simulink model "HWCOSIM_PHcontr_V2"  (R2020a)
settings: Solver=ode45  StartTime=0.0  StopTime=20  MaxStep=1e-5  RelTol=1e-3
undefined symbols (not defined in the file): A, den_loop_filtZ, f_step, fdesignblkfcn, FPGA_CLK, FPGA_Ts, Fref, G_loopfilt, gcbh, max_unwrap_periods, MECOS_cl_den, MECOS_MAX_PULSES, N, Nslits, num_loop_filtZ, PFD_noise_corrtime, PFD_Ts, phase_setpoint_degrees, PHCTRLR_CLK, PHCTRLR_Ts, Tref, unwrap_res_thr
libraries: dspsigops x5, simulink x4, dspmlti4 x4, simulink_extras x2, xbsIndex_r4 x1, dsparch4 x1, dspfdesign x1, JTAGRuntimeCosim_r4 x1
settings Model: Creator=valbas  LastModifiedBy=valbas
settings SolverCC: AlgebraicLoopSolver=LineSearch

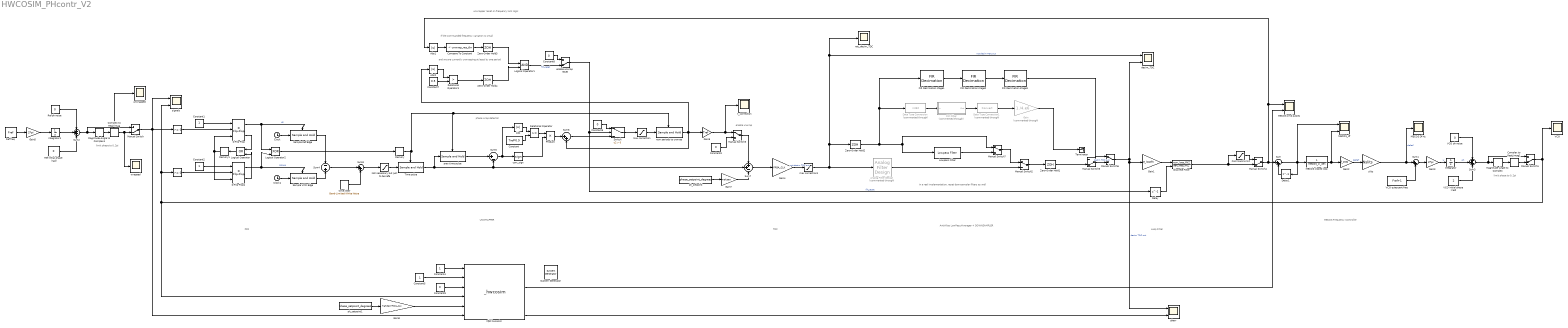
== system HWCOSIM_PHcontr_V2 ==
  note: enable unwrap
  note: in a real implementation, reset downsampler filters as well
  note: if the commanded frequency variation is small
  note: unwrapper reset on frequency lock logic
  note: phase wrap detector
  note: limit phase to 0..2pi
  note: TDC
  note: AntiAlias LowPass/Averager +
      | DOWNSAMPLER
  note: Loop Filter
  note: MECOS Frequency Controller
  note: limit phase to 0..2pi
  note: PFD
  note: UNWRAPPER
  note: and we are currently unwrapping at least by one period
  " " : simulink/Logic and Bit Operations/Compare To Constant  relop=>=  const=0  OutDataTypeStr=boolean
  "  " : simulink/Logic and Bit Operations/Compare To Constant  relop=>=  const=0  OutDataTypeStr=boolean
  " System Generator" : xbsIndex_r4/ System Generator  Tag=genX  xilinxfamily=zynq  part=xc7z020  speed=-1  package=clg484  synthesis_tool=Vivado  clock_wrapper=Clock Enables  directory=./netlist  proj_type=Vivado  Synth_file=Vivado Synthesis Defaults  Impl_file=Vivado Implementation Defaults  testbench=off  simulink_period=FPGA_Ts  sysclk_period=FPGA_Ts*1e9  dcm_input_clock_period=10  incr_netlist=off  trim_vbits=Everywhere in SubSystem  dbl_ovrd=According to Block Masks  core_generation=According to Block Masks  run_coregen=off  deprecated_control=off  eval_field=0  block_type=sysgen
  Abs : Abs
  Abs1 : Abs
  Abs2 : Abs
  Analog Filter Design : dsparch4/Analog Filter Design  Commented=through  method=Chebyshev II  filttype=Lowpass  N=8  Wlo=100  Whi=80  Rp=2  Rs=50
  CIC Filter : Subsystem  Commented=through  DialogController=fdesignblkfcn  InitFcn=fdesignblkfcn(gcbh, {'InitFcn'});  mask(CIC Filter){}
      mask help: Design a CIC filter
      settings: CopyFcn=fdesignblkfcn(gcbh, {'CopyFcn'});
      mask Help: helpview(mapfilelocation('dsp'), 'dspcicfilter');
      mask Display: disp('CIC')
  Clock : Clock
  Clock1 : Clock
  Command Limit : Saturate  UpperLimit=MECOS_MAX_PULSES/PHCTRLR_CLK  LowerLimit=-MECOS_MAX_PULSES/PHCTRLR_CLK
  Compare To Constant : simulink/Logic and Bit Operations/Compare To Constant  relop=<  const=unwrap_res_thr  OutDataTypeStr=boolean
  Complex to Real-Imag : ComplexToRealImag  Output=Real
  Complex to Real-Imag1 : ComplexToRealImag  Output=Real
  Constant : Constant  Value=Tref*0.9
  Constant{1..2,4..5} (4 alike) : Constant  OutDataTypeStr=boolean
  Constant3 : Constant  Value=0
  Constant6 : Constant  Value=0
  Constant7 : Constant  Value=0.5
  Constant8 : Constant  Value=0  OutDataTypeStr=boolean
  Constant9 : Constant  Value=0  OutDataTypeStr=boolean
  D Flip-Flop : simulink_extras/Flip Flops/D Flip-Flop
  D Flip-Flop1 : simulink_extras/Flip Flops/D Flip-Flop
  Data Type Conversion : DataTypeConversion  Commented=through  OutDataTypeStr=int32  RndMeth=Round
  Data Type Conversion1 : DataTypeConversion  Commented=through  RndMeth=Round
  Delay : Delay  DelayLength=1
  Delay1 : Delay  DelayLength=1
  Discrete Filter : DiscreteFilter  Numerator=num_loop_filtZ  Denominator=den_loop_filtZ  ExternalReset=Rising
      settings: InputPortMap=u0,r7
  FIR Decimation stage1 : dspmlti4/FIR Decimation  FilterSource=Dialog parameters  h=Num  D=10  filtStruct=Direct form  FilterObject=FDECIM  InputProcessing=Columns as channels (frame based)  framing=Allow multirate processing  inputOffset=0  outputBufInitCond=0  roundingMode=Floor  overflowMode=off  firstCoeffDataTypeStr=Inherit: Same word length as input  firstCoeffMin=[]  firstCoeffMax=[]  firstCoeffLastDataTypeStr=Inherit: Same word length as input  outputDataTypeStr=Inherit: Same as accumulator  outputMin=[]  outputMax=[]  outputLastDataTypeStr=Inherit: Same as accumulator
  FIR Decimation stage2 : dspmlti4/FIR Decimation  FilterSource=Dialog parameters  h=Num  D=10  filtStruct=Direct form  FilterObject=FDECIM  InputProcessing=Columns as channels (frame based)  framing=Allow multirate processing  inputOffset=0  outputBufInitCond=0  roundingMode=Floor  overflowMode=off  firstCoeffDataTypeStr=Inherit: Same word length as input  firstCoeffMin=[]  firstCoeffMax=[]  firstCoeffLastDataTypeStr=Inherit: Same word length as input  outputDataTypeStr=Inherit: Same as accumulator  outputMin=[]  outputMax=[]  outputLastDataTypeStr=Inherit: Same as accumulator
  FIR Decimation stage3 : dspmlti4/FIR Decimation  FilterSource=Dialog parameters  h=Num  D=10  filtStruct=Direct form  FilterObject=FDECIM  InputProcessing=Columns as channels (frame based)  framing=Allow multirate processing  inputOffset=0  outputBufInitCond=0  roundingMode=Floor  overflowMode=off  firstCoeffDataTypeStr=Inherit: Same word length as input  firstCoeffMin=[]  firstCoeffMax=[]  firstCoeffLastDataTypeStr=Inherit: Same word length as input  outputDataTypeStr=Inherit: Same as accumulator  outputMin=[]  outputMax=[]  outputLastDataTypeStr=Inherit: Same as accumulator
  Gain : Gain  Commented=through  Gain=1./4.e6
  Gain1 : Gain  Gain=G_loopfilt
  Gain2 : Gain  Gain=f_step
  Gain3 : Gain  Gain=2*pi
  Gain4 : Gain  Gain=FPGA_CLK
  Gain5 : Gain  Gain=2*pi
  Gain6 : Gain  Gain=Tref
  Gain7 : Gain  Gain=Tref/360
  Gain8 : Gain  Gain=Tref/360*FPGA_CLK
  Integrator : Integrator
  Integrator1 : Integrator
  Logical Operator : Logic  Operator=OR  IconShape=distinctive  AllPortsSameDT=off  OutDataTypeStr=boolean
  Logical Operator1 : Logic  IconShape=distinctive  AllPortsSameDT=off  OutDataTypeStr=boolean
  Logical Operator2 : Logic  Operator=XOR  IconShape=distinctive  AllPortsSameDT=off  OutDataTypeStr=boolean
  Lowpass Filter : dspfdesign/Lowpass Filter  FilterType=FIR  DesignForMinimumOrder=on  FilterOrder=50  PassbandFrequency=30  StopbandFrequency=70  PassbandRipple=1  StopbandAttenuation=30  InheritSampleRate=off  SampleRate=100e3  SimulateUsing=Interpreted execution  roundingMode=Floor  coeffsDataTypeStr=fixdt(1,16)
  MECOS Df Hz : Scope
  MECOS closed loop : TransferFcn  Denominator=MECOS_cl_den
  MECOS cmd pulses : Scope  NumInputPorts=2
  MECOS_df : Scope  NumInputPorts=2
  Magnitude-Angle to Complex : MagnitudeAngleToComplex  Input=Angle  ConstantPart=1
  Magnitude-Angle to Complex1 : MagnitudeAngleToComplex  Input=Angle  ConstantPart=1
  Manual Switch{,1,4..5} (4 alike) : ManualSwitch  CurrentSetting=0
  Manual Switch{2..3,6..7} (4 alike) : ManualSwitch
  Memory : Memory
  Memory1 : Memory
  Not necessary but just to be safe : Saturate  UpperLimit=Tref  LowerLimit=-Tref
  Product : Product
  Ref freq : Constant  Value=Fref
  Ref initial phase (rad) : Constant  Value=0
  Ref ph noise : Constant  Value=0
  Relational Operator : RelationalOperator  OutDataTypeStr=boolean  RndMeth=Simplest
  Relational Operator1 : RelationalOperator  Operator=>  OutDataTypeStr=boolean  RndMeth=Simplest
  Sample Ref Edge : dspsigops/Sample and Hold  trig=Rising edge  initCond=0  latchinput=on
  Sample VCO Edge : dspsigops/Sample and Hold  trig=Rising edge  initCond=0  latchinput=on
  Sum{,1,6,8} (4 alike) : Sum  Inputs=|++
  Sum2 : Sum  Inputs=+++
  Sum3 : Sum  Inputs=+++
  Sum4 : Sum  Inputs=-|+
  Sum5 : Sum  Inputs=|+-
  Sum7 : Sum  Inputs=++-
  Switch : Switch  Criteria=u2 > Threshold
  Terminator : Terminator
  Time pulse : dspsigops/Sample and Hold  trig=Falling edge  initCond=0  latchinput=on
  VCO : Scope
  VCO initial phase (rad) : Constant  Value=2
  VCO ph noise : Constant  Value=0
  VCO quiescent freq : Constant  Value=Fref+1
  Zero-Order Hold1 : ZeroOrderHold  SampleTime=PHCTRLR_Ts
  Zero-Order Hold2 : ZeroOrderHold  SampleTime=PFD_Ts
  Zero-Order Hold3 : ZeroOrderHold  SampleTime=PHCTRLR_Ts
  Zero-Order Hold4 : ZeroOrderHold  SampleTime=PHCTRLR_Ts
  corr_sign : Signum
  decim_TDC : Scope  NumInputPorts=2
  enable unwrap reset : ManualSwitch  CurrentSetting=0
  max correction : Saturate  UpperLimit=max_unwrap_periods  LowerLimit=-max_unwrap_periods
  max correction1 : Saturate  UpperLimit=max_unwrap_periods*Tref*FPGA_CLK  LowerLimit=-max_unwrap_periods*Tref*FPGA_CLK
  not_decim_TDC : Scope
  num periods to unwrap : dspsigops/Sample and Hold  trig=Falling edge  initCond=0  latchinput=on
  ph_setpoint : Constant  Value=phase_setpoint_degrees
  ph_setpoint1 : Constant  Value=phase_setpoint_degrees
  pherr : Scope  NumInputPorts=2
  prev time pulse : dspsigops/Sample and Hold  trig=Falling edge  initCond=0  latchinput=on
  signals : Scope  NumInputPorts=2
  slits : Gain  Gain=Nslits
  t_correction : Scope
  time jitter : simulink/Sources/Band-Limited White Noise  Cov=PFD_jitter_PSD  Ts=PFD_noise_corrtime  seed=[23341]
  unwrapped : Scope
  wrapped : Scope
  zfph hwcosim : JTAGRuntimeCosim_r4/_hwcosim  clkSrc=Single Stepped  hasCombinationalPath=on  bitfileName=C:\xilinxworks\netlist\zfph.bit  skipConfig=off  dispPartInfo=off  useZynqReconfigScript=on  cable=Auto Detect  speed=N/A  cablePort=N/A  cableLocation=Local  shareCable=off  design_xtable=|  engineDll=JTAGCosimEngine.dll  cableWaitTime=10  bscanPos=-1  IRLengths=[]  useWaitBox=1  hasBufgmux=on  Scheme=Cosim  useCmdProc=1  hasProc=0  useImpact=0  printLogFile=0  userChain=2  block_type=jtagcosim
      | {
      |     'clkWrapper' => 'zfph',
      |     'burstMode' => false,
      |     'burstFifoDepth' => '1024',
      |     'shared_memories' => {},
      |     'clocksGcd' => 1,
      |     'device' => {
      |       'family' => 'zynq',
      |       'part' => 'xc7z020',
      |       'package' => 'clg484',
      |       'speed' => '-1',
      |     },
      |     'ports' => {
      |       'unwr_reset_enable' => {
      |         'direction' => 'in',
      |         'width' => 1,
      |         'name' => 'unwr_reset_enable',
      |         'period' => 1,
      |         'icon_text' => 'unwr_reset_enable',
      |         'type' => 'Bool',
      |         'arithmetic_type' => 'xlUnsigned',
      |         'dat_file' => 'zfph_unwr_reset_enable.dat',
      |         'bin_pt' => 0,
      |         'addr_offset' => 0,
      |         'bd_port_index' => 0,
      |       },
      |       'unwr_en' => {
      |         'direction' => 'in',
      |         'width' => 1,
      |         'name' => 'unwr_en',
      |         'period' => 1,
      |         'icon_text' => 'unwr_en',
      |         'type' => 'Bool',
      |         'arithmetic_type' => 'xlUnsigned',
      |         'dat_file' => 'zfph_unwr_en.dat',
      |         'bin_pt' => 0,
      |         'addr_offset' => 4,
      |         'bd_port_index' => 1,
      |       },
      |       'reset' => {
      |         'direction' => 'in',
      |         'width' => 1,
      |         'name' => 'reset',
      |         'period' => 1,
      |         'icon_text' => 'reset',
      |         'type' => 'Bool',
      |         'arithmetic_type' => 'xlUnsigned',
      |         'dat_file' => 'zfph_reset.dat',
      |         'bin_pt' => 0,
      |         'addr_offset' => 8,
      |         'bd_port_index' => 2,
      |       },
      |       'vcoin' => {
      |         'direction' => 'in',
      |         'width' => 1,
      |         'name' => 'vcoin',
      |         'period' => 1,
      |         'icon_text' => 'VCOin',
      |         'type' => 'Bool',
      |         'arithmetic_type' => 'xlUnsigned',
      |         'dat_file' => 'zfph_vcoin.dat',
      |         'bin_pt' => 0,
      |         'addr_offset' => 12,
      |         'bd_port_index' => 3,
      |       },
      |       'setpoint_cnts' => {
      |         'direction' => 'in',
      |         'width' => 17,
      |         'name' => 'setpoint_cnts',
      |         'period' => 1,
      |         'icon_text' => 'Setpoint_cnts',
      |         'type' => 'Fix_17_0',
      |         'arithmetic_type' => 'xlSigned',
      |         'dat_file' => 'zfph_setpoint_cnts.dat',
      |         'bin_pt' => 0,
      |         'addr_offset' => 16,
      |         'bd_port_index' => 4,
      |       },
      |       'refin' => {
      |         'direction' => 'in',
      |         'width' => 1,
      |         'name' => 'refin',
      |         'period' => 1,
      |         'icon_text' => 'REFin',
      |         'type' => 'Bool',
      |         'arithmetic_type' => 'xlUnsigned',
      |         'dat_file' => 'zfph_refin.dat',
      |         'bin_pt' => 0,
      |         'addr_offset' => 20,
      |         'bd_port_index' => 5,
      |       },
      |       'dec_pulses' => {
      |         'direction' => 'out',
      |         'width' => 1,
      |         'name' => 'dec_pulses',
      |         'period' => 12500,
      |         'icon_text' => 'DEC_PULSES',
      |         'type' => 'Bool',
      |         'arithmetic_type' => 'xlUnsigned',
      |         'dat_file' => 'zfph_dec_pulses.dat',
      |         'bin_pt' => 0,
      |         'addr_offset' => 24,
      |         'bd_port_index' => 0,
      |       },
      |       'dec_pwm' => {
      |         'direction' => 'out',
      |         'width' => 1,
      |         'name' => 'dec_pwm',
      |         'period' => 12500,
      |         'icon_text' => 'DEC_PWM',
      |         'type' => 'Bool',
      |         'arithmetic_type' => 'xlUnsigned',
      |         'dat_file' => 'zfph_dec_pwm.dat',
      |         'bin_pt' => 0,
      |         'addr_offset' => 28,
      |         'bd_port_index' => 1,
      |       },
      |       'df_comm' => {
      |         'direction' => 'out',
      |         'width' => 22,
      |         'name' => 'df_comm',
      |         'period' => 1250000,
      |         'icon_text' => 'DF_COMM',
      |         'type' => 'Fix_22_0',
      |         'arithmetic_type' => 'xlSigned',
      |         'dat_file' => 'zfph_df_comm.dat',
      |         'bin_pt' => 0,
      |         'addr_offset' => 32,
      |         'bd_port_index' => 2,
      |       },
      |       'inc_pulses' => {
      |         'direction' => 'out',
      |         'width' => 1,
      |         'name' => 'inc_pulses',
      |         'period' => 12500,
      |         'icon_text' => 'INC_PULSES',
      |         'type' => 'Bool',
      |         'arithmetic_type' => 'xlUnsigned',
      |         'dat_file' => 'zfph_inc_pulses.dat',
      |         'bin_pt' => 0,
      |         'addr_offset' => 36,
      |         'bd_port_index' => 3,
      |       },
      |       'inc_pwm' => {
      |         'direction' => 'out',
      |         'width' => 1,
      |         'name' => 'inc_pwm',
      |         'period' => 12500,
      |         'icon_text' => 'INC_PWM',
      |         'type' => 'Bool',
      |         'arithmetic_type' => 'xlUnsigned',
      |         'dat_file' => 'zfph_inc_pwm.dat',
      |         'bin_pt' => 0,
      |         'addr_offset' => 40,
      |         'bd_port_index' => 4,
      |       },
      |       'ph_err' => {
      |         'direction' => 'out',
      |         'width' => 24,
      |         'name' => 'ph_err',
      |         'period' => 1250000,
      |         'icon_text' => 'PH_ERR',
      |         'type' => 'Fix_24_7',
      |         'arithmetic_type' => 'xlSigned',
      |         'dat_file' => 'zfph_ph_err.dat',
      |         'bin_pt' => 7,
      |         'addr_offset' => 44,
      |         'bd_port_index' => 5,
      |       },
      |     },
      |   }
  wires:
  Gain1/1 -> Discrete Filter/1
  Manual Switch6/1 -> decim_TDC/2, pherr/1, Gain1/1  "decim TDC out"
  Delay1/1 -> Sum/2
  Sum/1 -> Delay1/1, MECOS closed loop/1, MECOS_df/1
  MECOS closed loop/1 -> Gain2/1, MECOS_df/2
  slits/1 -> MECOS Df Hz/1, Sum1/1  "deltaf"
  VCO quiescent freq/1 -> Sum1/2
  Sum1/1 -> Gain3/1
  Gain3/1 -> Integrator/1  "w"
  Integrator/1 -> Sum3/2  "ph"
  Magnitude-Angle to Complex/1 -> Complex to Real-Imag1/1
  Magnitude-Angle to Complex1/1 -> Complex to Real-Imag/1
  Gain5/1 -> Integrator1/1
  Ref freq/1 -> Gain5/1
  VCO initial phase (rad)/1 -> Sum3/3
  Sum3/1 -> Manual Switch1/1, Magnitude-Angle to Complex/1
  Sum2/1 -> unwrapped/1, Manual Switch/1, Magnitude-Angle to Complex1/1
  Complex to Real-Imag/1 -> wrapped/1, Manual Switch/2
  max correction1/1 -> not_decim_TDC/1, decim_TDC/1, Zero-Order Hold2/1, Analog Filter Design/1  "not decim TDC out"
  Manual Switch/1 -> zfph hwcosim/6, signals/1, " "/1
  Complex to Real-Imag1/1 -> Manual Switch1/2
  Discrete Filter/1 -> Command Limit/1, Manual Switch4/2
  Lowpass Filter/1 -> Manual Switch7/2
  Analog Filter Design/1 -> Manual Switch2/2
  Manual Switch2/1 -> Zero-Order Hold1/1
  " "/1 -> D Flip-Flop/2
  Sample Ref Edge/1 -> Sum4/1
  "  "/1 -> D Flip-Flop1/2
  Manual Switch1/1 -> VCO/1, "  "/1, signals/2, zfph hwcosim/4
  Sample VCO Edge/1 -> Sum4/2
  Clock/1 -> Sample Ref Edge/1
  Clock1/1 -> Sample VCO Edge/1
  Sum4/1 -> Sum8/1
  Logical Operator2/1 -> Memory/1
  Logical Operator/1 -> Memory1/1
  D Flip-Flop1/2 -> Logical Operator/2
  Constant2/1 -> D Flip-Flop1/1
  Memory1/1 -> D Flip-Flop1/3, D Flip-Flop/3
  D Flip-Flop/2 -> Logical Operator/1
  Constant1/1 -> D Flip-Flop/1
  D Flip-Flop/1 -> Logical Operator2/1, Sample Ref Edge/Trigger  "UP"
  D Flip-Flop1/1 -> Logical Operator2/2, Sample VCO Edge/Trigger  "DOWN"
  Sum5/1 -> Abs/1, corr_sign/1
  Constant/1 -> Relational Operator/2
  Abs/1 -> Relational Operator/1
  num periods to unwrap/1 -> Sum6/2, Abs2/1, Gain6/1
  corr_sign/1 -> Product/2
  Sum6/1 -> Switch/3
  Gain6/1 -> t_correction/1, Manual Switch3/1
  Constant3/1 -> Manual Switch3/2
  Manual Switch3/1 -> Sum7/1
  prev time pulse/1 -> Sum5/1
  Time pulse/1 -> prev time pulse/1, Sum5/2, Sum7/2
  Command Limit/1 -> Manual Switch4/1
  Not necessary but just to be safe/1 -> Time pulse/1
  Data Type Conversion/1 -> CIC Filter/1(In)
  CIC Filter/1(Out) -> Data Type Conversion1/1
  Data Type Conversion1/1 -> Gain/1
  Zero-Order Hold1/1 -> Manual Switch5/2
  Gain/1 -> Terminator/1
  Manual Switch5/1 -> Manual Switch6/2  "decim TDC out"
  FIR Decimation stage1/1 -> FIR Decimation stage2/1
  FIR Decimation stage2/1 -> FIR Decimation stage3/1
  FIR Decimation stage3/1 -> Manual Switch6/1
  Integrator1/1 -> Sum2/2
  Ref initial phase (rad)/1 -> Sum2/3
  VCO ph noise/1 -> Sum3/1
  Manual Switch7/1 -> Manual Switch2/1
  Zero-Order Hold2/1 -> FIR Decimation stage1/1, Data Type Conversion/1, Manual Switch7/1, Lowpass Filter/1
  max correction/1 -> num periods to unwrap/1
  Sum7/1 -> Gain4/1
  Gain4/1 -> max correction1/1  "not decim TDC out"
  Ref ph noise/1 -> Sum2/1
  Switch/1 -> max correction/1
  Abs1/1 -> Compare To Constant/1
  Compare To Constant/1 -> Zero-Order Hold3/1
  Relational Operator/1 -> Product/1
  Product/1 -> Sum6/1
  Memory/1 -> Time pulse/Trigger, num periods to unwrap/Trigger, prev time pulse/Trigger
  Delay/1 -> Discrete Filter/2
  Constant7/1 -> Relational Operator1/2
  Relational Operator1/1 -> Zero-Order Hold4/1
  enable unwrap reset/1 -> Delay/1, Switch/2  "filt_reset"
  Manual Switch4/1 -> Abs1/1, MECOS cmd pulses/1, Sum/1
  Zero-Order Hold4/1 -> Logical Operator1/2
  Abs2/1 -> Relational Operator1/1
  Zero-Order Hold3/1 -> Logical Operator1/1
  Constant8/1 -> enable unwrap reset/1
  ph_setpoint/1 -> Gain7/1
  Gain7/1 -> Sum7/3
  Constant6/1 -> Switch/1
  Logical Operator1/1 -> enable unwrap reset/2  "filt_reset"
  Sum8/1 -> Not necessary but just to be safe/1
  time jitter/1 -> Sum8/2
  Gain2/1 -> slits/1  "deltaf"
  Constant4/1 -> zfph hwcosim/1
  Constant5/1 -> zfph hwcosim/2
  Constant9/1 -> zfph hwcosim/3
  ph_setpoint1/1 -> Gain8/1
  Gain8/1 -> zfph hwcosim/5
  zfph hwcosim/3 -> MECOS cmd pulses/2
  zfph hwcosim/6 -> pherr/2

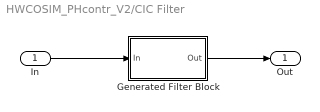
== system HWCOSIM_PHcontr_V2/CIC Filter ==
  In : Inport
  Generated Filter Block : Subsystem  Tag=BlockMethodSubSystem
  Out : Outport  VectorParamsAs1DForOutWhenUnconnected=off
  wires:
  In/1 -> Generated Filter Block/1(In)
  Generated Filter Block/1(Out) -> Out/1

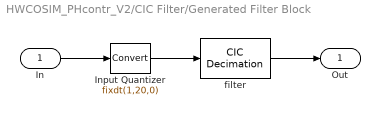
== system HWCOSIM_PHcontr_V2/CIC Filter/Generated Filter Block ==
  In : Inport
  Input Quantizer : DataTypeConversion  OutDataTypeStr=fixdt(1,20,0)  RndMeth=Round  SaturateOnIntegerOverflow=on
  filter : dspmlti4/CIC Decimation  filtFrom=Dialog parameters  filtobj=CICDECIM  ftype=Decimator  R=1000  M=2  N=2  filterInternals=Full precision  BPS=[42 42 42 42]  FLPS=[0 0 0 0]  outputWordLength=42  outputFracLength=0  launchFVT=off  framing=Maintain input frame rate  RateOptions=Allow multirate processing
      settings: SourceProductBaseCode=DS
  Out : Outport
  wires:
  In/1 -> Input Quantizer/1
  Input Quantizer/1 -> filter/1
  filter/1 -> Out/1
